simulink model "DCMotorOLACDC"  (R2018b)
settings: Solver=ode23tb  StartTime=0.0  StopTime=10  MaxStep=5e-5  MinStep=5e-7  RelTol=1e-3
InitFcn:
  | firing_angle1=30;
  | firing_angle2=45;
  | f=50;
  | T=1/f;
  | firing_delay1=(firing_angle1/360)*T;
  | firing_space=(60/360)*T;
  | firing_delay2=(firing_angle2/360)*T;
libraries: powerlib x10, powerlib_meascontrol x1, peThyristorSixPulseGenerator x1
settings Model: Creator=Koosha  LastModifiedBy=Koosha
settings SolverCC: ZeroCrossAlgorithm=Adaptive
settings DebuggingCC: IgnoredZcDiagnostic=none

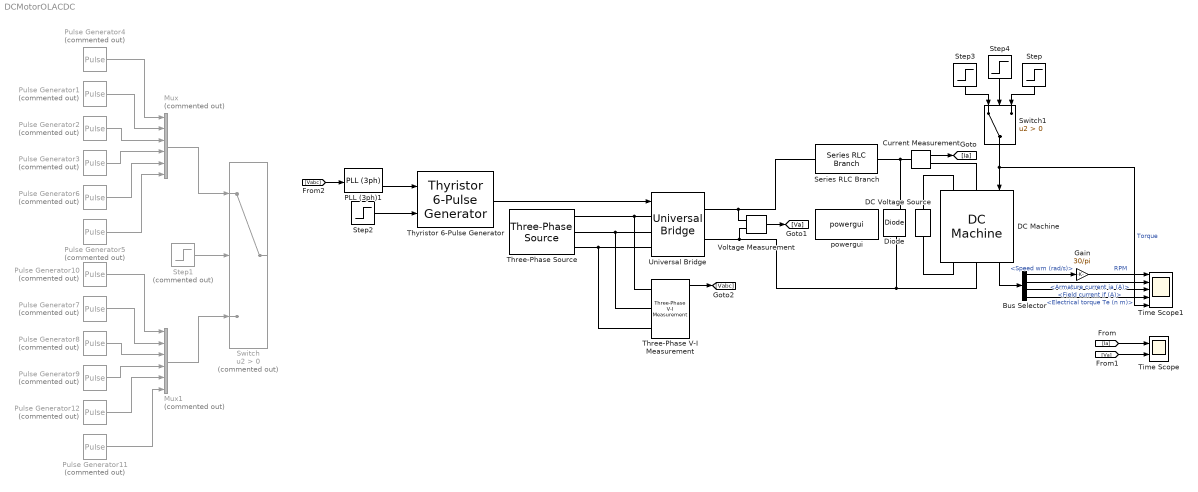
== system DCMotorOLACDC ==
  Bus Selector : BusSelector  OutputSignals=Speed wm (rad/s),Armature current ia (A),Field current if (A),Electrical torque Te (n m)
  Current Measurement : powerlib/Measurements/Current Measurement  PhasorSimulation=off  OutputType=Complex  PSBequivalent=0
  DC Machine : powerlib/Machines/DC Machine  PresetModel=03: 5HP 500V 1750RPM Field:300V  MechanicalLoad=Torque TL  FieldType=Wound  ShowDetailedParameters=on  MeasurementBus=off  RLa=[11.2 0.1215]  RLf=[281.3 156]  Laf=1.976  MachineConstant=Torque constant (N.m/A)  Ke=1.8  Kt=1.8  J=0.02215  Bm=0.002953  Tf=0.5161  w0=0  Ifinit=0  TsPowergui=0  TsBlock=-1
  DC Voltage Source : powerlib/Electrical Sources/DC Voltage Source  Amplitude=300  Measurements=Voltage
  Diode : powerlib/Power Electronics/Diode  Ron=0.001  Lon=0  Vf=0.8  IC=0  UseSnubber=0  Rs=500  Cs=250e-9  Measurements=on
  Gain : Gain  Gain=30/pi
  Mux : Mux  Commented=on  Inputs=6
  Mux1 : Mux  Commented=on  Inputs=6
  PLL (3ph)1 : powerlib_meascontrol/PLL/PLL (3ph)  Fmin=45  Par_Init=[0, 60]  ParK=[180, 3200, 1]  TcD=1e-4  MaxRateChangeFreq=12  FilterCutOffFreq=25  Ts=0  AGC=on
  Pulse Generator1 : DiscretePulseGenerator  Commented=on  PulseType=Time based  Period=0.02  PulseWidth=5  PhaseDelay=firing_delay1+firing_space
  Pulse Generator10 : DiscretePulseGenerator  Commented=on  PulseType=Time based  Period=0.02  PulseWidth=5  PhaseDelay=firing_delay2
  Pulse Generator11 : DiscretePulseGenerator  Commented=on  PulseType=Time based  Period=0.02  PulseWidth=5  PhaseDelay=firing_delay2+(5*firing_space)
  Pulse Generator12 : DiscretePulseGenerator  Commented=on  PulseType=Time based  Period=0.02  PulseWidth=5  PhaseDelay=firing_delay2+(4*firing_space)
  Pulse Generator2 : DiscretePulseGenerator  Commented=on  PulseType=Time based  Period=0.02  PulseWidth=5  PhaseDelay=firing_delay1+(2*firing_space)
  Pulse Generator3 : DiscretePulseGenerator  Commented=on  PulseType=Time based  Period=0.02  PulseWidth=5  PhaseDelay=firing_delay1+(3*firing_space)
  Pulse Generator4 : DiscretePulseGenerator  Commented=on  PulseType=Time based  Period=0.02  PulseWidth=5  PhaseDelay=firing_delay1
  Pulse Generator5 : DiscretePulseGenerator  Commented=on  PulseType=Time based  Period=0.02  PulseWidth=5  PhaseDelay=firing_delay1+(5*firing_space)
  Pulse Generator6 : DiscretePulseGenerator  Commented=on  PulseType=Time based  Period=0.02  PulseWidth=5  PhaseDelay=firing_delay1+(4*firing_space)
  Pulse Generator7 : DiscretePulseGenerator  Commented=on  PulseType=Time based  Period=0.02  PulseWidth=5  PhaseDelay=firing_delay2+firing_space
  Pulse Generator8 : DiscretePulseGenerator  Commented=on  PulseType=Time based  Period=0.02  PulseWidth=5  PhaseDelay=firing_delay2+(2*firing_space)
  Pulse Generator9 : DiscretePulseGenerator  Commented=on  PulseType=Time based  Period=0.02  PulseWidth=5  PhaseDelay=firing_delay2+(3*firing_space)
  Series RLC Branch : powerlib/Elements/Series RLC Branch  LConnTagsString=__new0  RConnTagsString=__new0  BranchType=L  Resistance=20  Inductance=1e-6  SetiL0=off  InitialCurrent=0  Capacitance=1e-6  Setx0=off  InitialVoltage=0  Measurements=None
  Step : Step  Time=3  Before=10  After=20  SampleTime=0
  Step1 : Step  Commented=on  Time=0.5  SampleTime=0
  Step2 : Step  Time=5  Before=pi/3  After=pi/6  SampleTime=0
  Step3 : Step  Time=7  Before=20  After=10  SampleTime=0
  Step4 : Step  Time=3  SampleTime=0
  Switch : Switch  Commented=on  Criteria=u2 > Threshold
  Switch1 : Switch  Criteria=u2 > Threshold
  Three-Phase V-I Measurement : powerlib/Measurements/Three-Phase V-I Measurement  VoltageMeasurement=phase-to-phase  SetLabelV=off  LabelV=Vabc  Vpu=off  VpuLL=off  CurrentMeasurement=yes  SetLabelI=off  LabelI=Iabc  Ipu=off  Pbase=100e6  Vbase=500e3  OutputType=Complex  PhasorSimulation=off  PSBequivalent=0
  Three-Phase Source : powerlib/Electrical Sources/Three-Phase Source  InternalConnection=Yg  VoltagePhases=off  Voltage=370  PhaseAngle=0  Voltage_phases=[25e3 25e3 25e3]/sqrt(3)  PhaseAngles_phases=[0 -120 +120]  Frequency=50  NonIdealSource=off  SpecifyImpedance=off  Resistance=0.01  Inductance=0  ShortCircuitLevel=100e6  BaseVoltage=25e3  XRratio=7  BusType=swing  Pref=10e3  Qref=0  Prefabc=[10e3, 10e3, 10e3]  Qrefabc=[0, 0, 0]  Qmin=-inf  Qmax=inf
  Thyristor 6-Pulse Generator : peThyristorSixPulseGenerator/Thyristor 6-Pulse Generator  Ord=Natural order of commutation  Pw=0.2  Ts=1e-5
  Time Scope : Scope  NumInputPorts=2
  Time Scope1 : Scope  NumInputPorts=5
  Universal Bridge : powerlib/Power Electronics/Universal Bridge  Arms=3  SnubberResistance=1e3  SnubberCapacitance=1e-6  Device=Thyristors  Ron=1e-3  Lon=0  ForwardVoltages="[  0  0  ]"  ForwardVoltage=0  GTOparameters=[ 10e-6 , 20e-6 ]  IGBTparameters=[ 1e-6 , 2e-6 ]  Measurements=None  Measurements_2=None  converterType=Rectifier
  Voltage Measurement : powerlib/Measurements/Voltage Measurement  PhasorSimulation=off  OutputType=Complex  PSBequivalent=0
  powergui : powerlib/powergui  Priority=1  SimulationMode=Discrete  SampleTime=5e-5  frequency=60  Iterations=50  frequencyindice=0  Pbase=100e6  ErrMax=1e-4  UnitsV=kV  UnitsW=MW  buscounter=0  FunctionMessages=on  echomessages=off  EnableUseOfTLC=off  CurrentSourceSwitches=off  DisableSnubberDevices=off  DisableRonSwitches=off  DisableVfSwitches=off  DisplayEquations=off  SolverType=Tustin/Backward Euler (TBE)  Interpol=off  ExternalGateDelay=off  methode=off  Ts=100  x0status=blocks  SPID=off  SwTol=0  HookPort=off  RestoreLinks=warning  ResistiveCurrentMeasurement=off  Frange=[0:2:500]  Ylog=off  Xlog=on  ShowGrid=off  save=off  variable=ZData  structure=0  ZoomFFT=off  StartTime=0.0  cycles=1  DisplayStyle=1  fundamental=60  FreqAxis=off  MaxFrequency=1000  frequencyindicesteady=1  RmsSteady=1  display=off
  wires:
  Current Measurement/1 -> [Ia]
  Voltage Measurement/1 -> [Va]
  Pulse Generator2/1 -> Mux/3
  Pulse Generator3/1 -> Mux/4
  Pulse Generator6/1 -> Mux/5
  Pulse Generator5/1 -> Mux/6
  Pulse Generator1/1 -> Mux/2
  Pulse Generator4/1 -> Mux/1
  DC Machine/1 -> Bus Selector/1
  Bus Selector/2 -> Time Scope1/2  "<Armature current ia (A)>"
  Bus Selector/3 -> Time Scope1/3  "<Field current if (A)>"
  Bus Selector/4 -> Time Scope1/4  "<Electrical torque Te (n m)>"
  [Ia] -> Time Scope/1
  [Va] -> Time Scope/2
  Pulse Generator9/1 -> Mux1/4
  Pulse Generator7/1 -> Mux1/2
  Pulse Generator12/1 -> Mux1/5
  Pulse Generator11/1 -> Mux1/6
  Pulse Generator10/1 -> Mux1/1
  Pulse Generator8/1 -> Mux1/3
  Mux/1 -> Switch/1
  Mux1/1 -> Switch/3
  Step1/1 -> Switch/2
  Three-Phase V-I Measurement/1 -> [Vabc]
  Thyristor 6-Pulse Generator/1 -> Universal Bridge/1
  [Vabc] -> PLL (3ph)1/1
  PLL (3ph)1/2 -> Thyristor 6-Pulse Generator/1
  Step2/1 -> Thyristor 6-Pulse Generator/2
  Step4/1 -> Switch1/2
  Step/1 -> Switch1/3
  Step3/1 -> Switch1/1
  Switch1/1 -> DC Machine/1, Time Scope1/5  "Torque"
  Bus Selector/1 -> Gain/1  "<Speed wm (rad/s)>"
  Gain/1 -> Time Scope1/1  "RPM"
  connections:
  Three-Phase Source/RConn1 -- Three-Phase V-I Measurement/LConn1 -- Universal Bridge/LConn1
  DC Voltage Source/RConn1 -- DC Machine/LConn2
  DC Voltage Source/LConn1 -- DC Machine/RConn2
  Three-Phase Source/RConn2 -- Three-Phase V-I Measurement/LConn2 -- Universal Bridge/LConn2
  Three-Phase Source/RConn3 -- Three-Phase V-I Measurement/LConn3 -- Universal Bridge/LConn3
  Series RLC Branch/LConn1 -- Universal Bridge/RConn1 -- Voltage Measurement/LConn1
  Current Measurement/LConn1 -- Series RLC Branch/RConn1 -- Diode/RConn1
  Diode/LConn1 -- Universal Bridge/RConn2 -- Voltage Measurement/LConn2 -- DC Machine/RConn1
  Current Measurement/RConn1 -- DC Machine/LConn1
